simulink model "IEEE123_4subsystem"  (R2022b)
settings: Solver=ode4  StartTime=0.0  StopTime=inf  FixedStep=Ts  MaxStep=1e-4  RelTol=1e-3
PreLoadFcn:
  | Ts = 50e-6;
PostLoadFcn:
  | Ts = 50e-6;
InitFcn:
  | %%%%%%%%%%%%%%%%%%%%%%%%
  | % Simulation data for the IEEE 123 Node Test Feeder model
  | %%%%%%%%%%%%%%%%%%%%%%%
  | 
  | % miles/km
  | mi2km = 1.60934;
  | 
  | % feet to km
  | ft2km = 0.0003048;
  | 
  | % microsiemens to Farads
  | ms2F = 1/2/pi/60*1e-6;
  | 
  | %% Configuration 1 - series reactance - ohm/mile
  | 
  | R_1 = [0.4576 0.1560 0.1535;0.1560 0.4666 0.1580;0.1535 0.1580 0.4615];
  | X_1 = [1.0780 0.5017 0.3849;0.5017 1.0482 0.4236;0.3849 0.4236 1.0651];
  | 
  | % charging susceptance - microsiemens/mile
  | 
  | B_1 = [5.6765 -1.8319 -0.6982;-1.8319 5.9809 -1.1645;-0.6982 -1.1645 5.3971];
  | 
  | % convert for SPS
  | 
  | R_1 = R_1/mi2km;
  | 
  | Rs_1=(R_1(1,1)+R_1(2,2)+R_1(3,3))/3;
  | Rm_1=(R_1(1,2)+R_1(1,3)+R_1(2,3))/3;
  | R1_1=Rs_1-Rm_1;
  | R0_1=Rs_1+2*Rm_1;
  | 
  | L_1 = X_1/mi2km/2/pi/60;
  | 
  | Ls_1=(L_1(1,1)+L_1(2,2)+L_1(3,3))/3;
  | Lm_1=(L_1(1,2)+L_1(1,3)+L_1(2,3))/3;
  | L1_1=Ls_1-Lm_1;
  | L0_1=Ls_1+2*Lm_1;
  | 
  | C_1 = B_1/mi2km*ms2F;
  | 
  | Cs_1=(C_1(1,1)+C_1(2,2)+C_1(3,3))/3;
  | Cm_1=(C_1(1,2)+C_1(1,3)+C_1(2,3))/3;
  | C1_1=Cs_1-Cm_1;
  | C0_1=Cs_1+2*Cm_1;
  | 
  | 
  | %% Configuration 2 - series reactance - ohm/mile
  | 
  | R_2 = [0.4666 0.1580 0.1560;0.1580 0.4615 0.1535;0.1560 0.1535 0.4576];
  | X_2 = [1.0482 0.4236 0.5017;0.4236 1.0651 0.3849;0.5017 0.3849 1.0780];
  | 
  | % charging susceptance - microsiemens/mile
  | 
  | B_2 = [5.9809 -1.1645 -1.8319;-1.1645 5.3971 -0.6982;-1.8319 -0.6982 5.6765];
  | 
  | % convert for SPS
  | 
  | R_2 = R_2/mi2km;
  | 
  | Rs_2=(R_2(1,1)+R_2(2,2)+R_2(3,3))/3;
  | ... (+341 lines)
undefined symbols (not defined in the file): D1, Delta, find_system, I, Left, MOV_segment9, powergui, Right, type, V, X
libraries: spsGroundLib x242, spsThreePhaseVIMeasurementLib x134, spsSeriesRLCBranchLib x107, spsSeriesRLCLoadLib x83, spsPiSectionLineLib x61, spsThreePhasePISectionLineLib x60, spsVoltageMeasurementLib x52, spsDCVoltageSourceLib x36, ssn_lib x28, artemis x24, spsACCurrentSourceLib x18, spsOnDelayLib x18
(part 3 of 15)

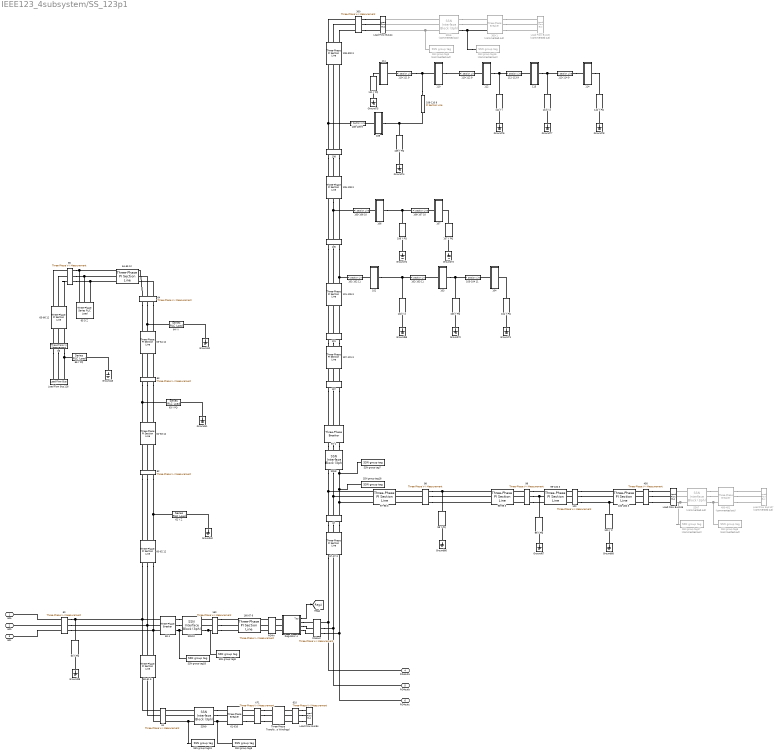
== system IEEE123_4subsystem/SS_123p1 ==
  100 : spsThreePhaseVIMeasurementLib/Three-Phase V-I Measurement  VoltageMeasurement=phase-to-ground  SetLabelV=on  LabelV=V100  Vpu=off  VpuLL=off  CurrentMeasurement=no  SetLabelI=on  LabelI=I65  Ipu=off  Pbase=100e6  Vbase=24900  OutputType=Complex  PhasorSimulation=off  PSBequivalent=0
  100 Y Z : spsSeriesRLCLoadLib/Series RLC Load  LConnTagsString=a  RConnTagsString=__new0  NominalVoltage=1.0*2401.78  NominalFrequency=60  ActivePower=40e3  InductivePower=20e3  CapacitivePower=0  Setx0=off  InitialVoltage=0  SetiL0=off  InitialCurrent=0  Measurements=None  LoadType=constant Z
  100-450 3 : spsThreePhasePISectionLineLib/Three-Phase PI Section Line  LConnTagsString=a|b|c  RConnTagsString=A|B|C  Length=800*ft2km  Frequency=60  Resistances=[R1_3 R0_3]  Inductances=[L1_3 L0_3]  Capacitances=[C1_3 C0_3]
  101 : spsThreePhaseVIMeasurementLib/Three-Phase V-I Measurement  VoltageMeasurement=phase-to-ground  SetLabelV=on  LabelV=V101  Vpu=off  VpuLL=off  CurrentMeasurement=no  SetLabelI=on  LabelI=I65  Ipu=off  Pbase=100e6  Vbase=24900  OutputType=Complex  PhasorSimulation=off  PSBequivalent=0
  101-102 11 : spsPiSectionLineLib/Pi Section Line  LConnTagsString=__new0  RConnTagsString=__new0  Phases=1  PiSections=1  Length=225*ft2km  Frequency=60  Resistance=R1_11  Inductance=L1_11  Capacitance=C1_11  SpecifyConductance=off  Conductance=0  Measurements=None  Measurements2=None
      settings: LibrarySourceBlock=sps_lib/Power Grid Elements/Pi Section Line
  101-105 3 : spsThreePhasePISectionLineLib/Three-Phase PI Section Line  LConnTagsString=a|b|c  RConnTagsString=A|B|C  Length=275*ft2km  Frequency=60  Resistances=[R1_3 R0_3]  Inductances=[L1_3 L0_3]  Capacitances=[C1_3 C0_3]
  102 : Subsystem
  102 Y Z : spsSeriesRLCLoadLib/Series RLC Load  LConnTagsString=a  RConnTagsString=__new0  NominalVoltage=1.0*2401.78  NominalFrequency=60  ActivePower=20e3  InductivePower=10e3  CapacitivePower=0  Setx0=off  InitialVoltage=0  SetiL0=off  InitialCurrent=0  Measurements=None  LoadType=constant Z
  102-103 11 : spsPiSectionLineLib/Pi Section Line  LConnTagsString=__new0  RConnTagsString=__new0  Phases=1  PiSections=1  Length=325*ft2km  Frequency=60  Resistance=R1_11  Inductance=L1_11  Capacitance=C1_11  SpecifyConductance=off  Conductance=0  Measurements=None  Measurements2=None
      settings: LibrarySourceBlock=sps_lib/Power Grid Elements/Pi Section Line
  103 : Subsystem
  103 Y PQ : spsSeriesRLCLoadLib/Series RLC Load  LConnTagsString=a  RConnTagsString=__new0  NominalVoltage=1.0*2401.78  NominalFrequency=60  ActivePower=40e3  InductivePower=20e3  CapacitivePower=0  Setx0=off  InitialVoltage=0  SetiL0=off  InitialCurrent=0  Measurements=None  LoadType=constant PQ
  103-104 11 : spsPiSectionLineLib/Pi Section Line  LConnTagsString=__new0  RConnTagsString=__new0  Phases=1  PiSections=1  Length=700*ft2km  Frequency=60  Resistance=R1_11  Inductance=L1_11  Capacitance=C1_11  SpecifyConductance=off  Conductance=0  Measurements=None  Measurements2=None
      settings: LibrarySourceBlock=sps_lib/Power Grid Elements/Pi Section Line
  104 : Subsystem
  104 Y PQ : spsSeriesRLCLoadLib/Series RLC Load  LConnTagsString=a  RConnTagsString=__new0  NominalVoltage=1.0*2401.78  NominalFrequency=60  ActivePower=40e3  InductivePower=20e3  CapacitivePower=0  Setx0=off  InitialVoltage=0  SetiL0=off  InitialCurrent=0  Measurements=None  LoadType=constant PQ
  105 : spsThreePhaseVIMeasurementLib/Three-Phase V-I Measurement  VoltageMeasurement=phase-to-ground  SetLabelV=on  LabelV=V105  Vpu=off  VpuLL=off  CurrentMeasurement=no  SetLabelI=on  LabelI=I65  Ipu=off  Pbase=100e6  Vbase=24900  OutputType=Complex  PhasorSimulation=off  PSBequivalent=0
  105-106 10 : spsPiSectionLineLib/Pi Section Line  LConnTagsString=__new0  RConnTagsString=__new0  Phases=1  PiSections=1  Length=225*ft2km  Frequency=60  Resistance=R1_10  Inductance=L1_10  Capacitance=C1_10  SpecifyConductance=off  Conductance=0  Measurements=None  Measurements2=None
      settings: LibrarySourceBlock=sps_lib/Power Grid Elements/Pi Section Line
  105-108 3 : spsThreePhasePISectionLineLib/Three-Phase PI Section Line  LConnTagsString=a|b|c  RConnTagsString=A|B|C  Length=325*ft2km  Frequency=60  Resistances=[R1_3 R0_3]  Inductances=[L1_3 L0_3]  Capacitances=[C1_3 C0_3]
  106 : Subsystem
  106 Y PQ : spsSeriesRLCLoadLib/Series RLC Load  LConnTagsString=a  RConnTagsString=__new0  NominalVoltage=1.0*2401.78  NominalFrequency=60  ActivePower=40e3  InductivePower=20e3  CapacitivePower=0  Setx0=off  InitialVoltage=0  SetiL0=off  InitialCurrent=0  Measurements=None  LoadType=constant PQ
  106-107 10 : spsPiSectionLineLib/Pi Section Line  LConnTagsString=__new0  RConnTagsString=__new0  Phases=1  PiSections=1  Length=575*ft2km  Frequency=60  Resistance=R1_10  Inductance=L1_10  Capacitance=C1_10  SpecifyConductance=off  Conductance=0  Measurements=None  Measurements2=None
      settings: LibrarySourceBlock=sps_lib/Power Grid Elements/Pi Section Line
  107 : Subsystem
  107 Y PQ : spsSeriesRLCLoadLib/Series RLC Load  LConnTagsString=a  RConnTagsString=__new0  NominalVoltage=1.0*2401.78  NominalFrequency=60  ActivePower=40e3  InductivePower=20e3  CapacitivePower=0  Setx0=off  InitialVoltage=0  SetiL0=off  InitialCurrent=0  Measurements=None  LoadType=constant PQ
  108 : spsThreePhaseVIMeasurementLib/Three-Phase V-I Measurement  VoltageMeasurement=phase-to-ground  SetLabelV=on  LabelV=V108  Vpu=off  VpuLL=off  CurrentMeasurement=no  SetLabelI=on  LabelI=I65  Ipu=off  Pbase=100e6  Vbase=24900  OutputType=Complex  PhasorSimulation=off  PSBequivalent=0
  108-109 9 : spsPiSectionLineLib/Pi Section Line  LConnTagsString=__new0  RConnTagsString=__new0  Phases=1  PiSections=1  Length=450*ft2km  Frequency=60  Resistance=R1_9  Inductance=L1_9  Capacitance=C1_9  SpecifyConductance=off  Conductance=0  Measurements=None  Measurements2=None
      settings: LibrarySourceBlock=sps_lib/Power Grid Elements/Pi Section Line
  108-300 3 : spsThreePhasePISectionLineLib/Three-Phase PI Section Line  LConnTagsString=a|b|c  RConnTagsString=A|B|C  Length=1000*ft2km  Frequency=60  Resistances=[R1_3 R0_3]  Inductances=[L1_3 L0_3]  Capacitances=[C1_3 C0_3]
  109 : Subsystem
  109 Y PQ : spsSeriesRLCLoadLib/Series RLC Load  LConnTagsString=a  RConnTagsString=__new0  NominalVoltage=1.0*2401.78  NominalFrequency=60  ActivePower=40e3  InductivePower=20e3  CapacitivePower=0  Setx0=off  InitialVoltage=0  SetiL0=off  InitialCurrent=0  Measurements=None  LoadType=constant PQ
  109-110 9 : spsPiSectionLineLib/Pi Section Line  LConnTagsString=__new0  RConnTagsString=__new0  Phases=1  PiSections=1  Length=300*ft2km  Frequency=60  Resistance=R1_9  Inductance=L1_9  Capacitance=C1_9  SpecifyConductance=off  Conductance=0  Measurements=None  Measurements2=None
      settings: LibrarySourceBlock=sps_lib/Power Grid Elements/Pi Section Line
  110 : Subsystem
  110-111 9 : spsPiSectionLineLib/Pi Section Line  LConnTagsString=__new0  RConnTagsString=__new0  Phases=1  PiSections=1  Length=575*ft2km  Frequency=60  Resistance=R1_9  Inductance=L1_9  Capacitance=C1_9  SpecifyConductance=off  Conductance=0  Measurements=None  Measurements2=None
      settings: LibrarySourceBlock=sps_lib/Power Grid Elements/Pi Section Line
  110-112 9 : spsPiSectionLineLib/Pi Section Line  LConnTagsString=__new0  RConnTagsString=__new0  Phases=1  PiSections=1  Length=125*ft2km  Frequency=60  Resistance=R1_9  Inductance=L1_9  Capacitance=C1_9  SpecifyConductance=off  Conductance=0  Measurements=None  Measurements2=None
      settings: LibrarySourceBlock=sps_lib/Power Grid Elements/Pi Section Line
  111 : Subsystem
  111 Y PQ : spsSeriesRLCLoadLib/Series RLC Load  LConnTagsString=a  RConnTagsString=__new0  NominalVoltage=1.0*2401.78  NominalFrequency=60  ActivePower=20e3  InductivePower=10e3  CapacitivePower=0  Setx0=off  InitialVoltage=0  SetiL0=off  InitialCurrent=0  Measurements=None  LoadType=constant PQ
  112 : Subsystem
  112 Y I : spsSeriesRLCLoadLib/Series RLC Load  LConnTagsString=a  RConnTagsString=__new0  NominalVoltage=1.0*2401.78  NominalFrequency=60  ActivePower=20e3  InductivePower=10e3  CapacitivePower=0  Setx0=off  InitialVoltage=0  SetiL0=off  InitialCurrent=0  Measurements=None  LoadType=constant I
  112-113 9 : spsPiSectionLineLib/Pi Section Line  LConnTagsString=__new0  RConnTagsString=__new0  Phases=1  PiSections=1  Length=525*ft2km  Frequency=60  Resistance=R1_9  Inductance=L1_9  Capacitance=C1_9  SpecifyConductance=off  Conductance=0  Measurements=None  Measurements2=None
      settings: LibrarySourceBlock=sps_lib/Power Grid Elements/Pi Section Line
  113 : Subsystem
  113 Y Z : spsSeriesRLCLoadLib/Series RLC Load  LConnTagsString=a  RConnTagsString=__new0  NominalVoltage=1.0*2401.78  NominalFrequency=60  ActivePower=40e3  InductivePower=20e3  CapacitivePower=0  Setx0=off  InitialVoltage=0  SetiL0=off  InitialCurrent=0  Measurements=None  LoadType=constant PQ
  113-114 9 : spsPiSectionLineLib/Pi Section Line  LConnTagsString=__new0  RConnTagsString=__new0  Phases=1  PiSections=1  Length=325*ft2km  Frequency=60  Resistance=R1_9  Inductance=L1_9  Capacitance=C1_9  SpecifyConductance=off  Conductance=0  Measurements=None  Measurements2=None
      settings: LibrarySourceBlock=sps_lib/Power Grid Elements/Pi Section Line
  114 : Subsystem
  142 Y PQ : spsSeriesRLCLoadLib/Series RLC Load  LConnTagsString=a  RConnTagsString=__new0  NominalVoltage=1.0*2401.78  NominalFrequency=60  ActivePower=20e3  InductivePower=10e3  CapacitivePower=0  Setx0=off  InitialVoltage=0  SetiL0=off  InitialCurrent=0  Measurements=None  LoadType=constant PQ
  160 : spsThreePhaseVIMeasurementLib/Three-Phase V-I Measurement  VoltageMeasurement=phase-to-ground  SetLabelV=on  LabelV=V160  Vpu=off  VpuLL=off  CurrentMeasurement=no  SetLabelI=on  LabelI=I160  Ipu=off  Pbase=100e6  Vbase=24900  OutputType=Complex  PhasorSimulation=off  PSBequivalent=0
  160 67 6 : spsThreePhasePISectionLineLib/Three-Phase PI Section Line  LConnTagsString=a|b|c  RConnTagsString=A|B|C  Length=350*ft2km  Frequency=60  Resistances=[R1_6 R0_6]  Inductances=[L1_6 L0_6]  Capacitances=[C1_6 C0_6]
  197 : spsThreePhaseVIMeasurementLib/Three-Phase V-I Measurement  VoltageMeasurement=phase-to-ground  SetLabelV=on  LabelV=V197  Vpu=off  VpuLL=off  CurrentMeasurement=no  SetLabelI=on  LabelI=I65  Ipu=off  Pbase=100e6  Vbase=24900  OutputType=Complex  PhasorSimulation=off  PSBequivalent=0
  197-101 3 : spsThreePhasePISectionLineLib/Three-Phase PI Section Line  LConnTagsString=a|b|c  RConnTagsString=A|B|C  Length=250*ft2km  Frequency=60  Resistances=[R1_3 R0_3]  Inductances=[L1_3 L0_3]  Capacitances=[C1_3 C0_3]
  300 : spsThreePhaseVIMeasurementLib/Three-Phase V-I Measurement  VoltageMeasurement=phase-to-ground  SetLabelV=on  LabelV=V300  Vpu=off  VpuLL=off  CurrentMeasurement=no  SetLabelI=on  LabelI=I65  Ipu=off  Pbase=100e6  Vbase=24900  OutputType=Complex  PhasorSimulation=off  PSBequivalent=0
  300-1 : spsThreePhaseBreakerLib/Three-Phase Breaker  Commented=on  InitialState=open  SwitchA=on  SwitchB=on  SwitchC=on  SwitchTimes="[1/60  5/60]"  External=off  BreakerResistance=0.01  SnubberResistance=1e6  SnubberCapacitance=inf  Measurements=None
  450 : spsThreePhaseVIMeasurementLib/Three-Phase V-I Measurement  VoltageMeasurement=phase-to-ground  SetLabelV=on  LabelV=V450  Vpu=off  VpuLL=off  CurrentMeasurement=no  SetLabelI=on  LabelI=I65  Ipu=off  Pbase=100e6  Vbase=24900  OutputType=Complex  PhasorSimulation=off  PSBequivalent=0
  450-451 : spsThreePhaseBreakerLib/Three-Phase Breaker  Commented=on  InitialState=open  SwitchA=on  SwitchB=on  SwitchC=on  SwitchTimes="[1/60  5/60]"  External=off  BreakerResistance=0.01  SnubberResistance=1e6  SnubberCapacitance=inf  Measurements=None
  60 : spsThreePhaseVIMeasurementLib/Three-Phase V-I Measurement  VoltageMeasurement=phase-to-ground  SetLabelV=on  LabelV=V60  Vpu=off  VpuLL=off  CurrentMeasurement=yes  SetLabelI=on  LabelI=I60  Ipu=off  Pbase=100e6  Vbase=24900  OutputType=Complex  PhasorSimulation=off  PSBequivalent=0
  60 Y PQ : spsSeriesRLCLoadLib/Series RLC Load  LConnTagsString=a  RConnTagsString=__new0  NominalVoltage=1.0*2401.78  NominalFrequency=60  ActivePower=20e3  InductivePower=10e3  CapacitivePower=0  Setx0=off  InitialVoltage=0  SetiL0=off  InitialCurrent=0  Measurements=None  LoadType=constant PQ
  60-1 : spsThreePhaseBreakerLib/Three-Phase Breaker  InitialState=closed  SwitchA=on  SwitchB=on  SwitchC=on  SwitchTimes="[1/60  5/60]"  External=off  BreakerResistance=0.01  SnubberResistance=1e6  SnubberCapacitance=inf  Measurements=None
  60-61 5 : spsThreePhasePISectionLineLib/Three-Phase PI Section Line  LConnTagsString=a|b|c  RConnTagsString=A|B|C  Length=550*ft2km  Frequency=60  Resistances=[R1_5 R0_5]  Inductances=[L1_5 L0_5]  Capacitances=[C1_5 C0_5]
  60-62 12 : spsThreePhasePISectionLineLib/Three-Phase PI Section Line  LConnTagsString=a|b|c  RConnTagsString=A|B|C  Length=250*ft2km  Frequency=60  Resistances=[R1_12 R0_12]  Inductances=[L1_12 L0_12]  Capacitances=[C1_12 C0_12]
  61 : spsThreePhaseVIMeasurementLib/Three-Phase V-I Measurement  VoltageMeasurement=phase-to-ground  SetLabelV=on  LabelV=V61  Vpu=off  VpuLL=off  CurrentMeasurement=no  SetLabelI=on  LabelI=I65  Ipu=off  Pbase=100e6  Vbase=24900  OutputType=Complex  PhasorSimulation=off  PSBequivalent=0
  61-610 : spsThreePhaseBreakerLib/Three-Phase Breaker  InitialState=closed  SwitchA=on  SwitchB=on  SwitchC=on  SwitchTimes="[1/60  5/60]"  External=off  BreakerResistance=0.01  SnubberResistance=1e6  SnubberCapacitance=inf  Measurements=None
  610 : spsThreePhaseVIMeasurementLib/Three-Phase V-I Measurement  VoltageMeasurement=phase-to-phase  SetLabelV=on  LabelV=V610  Vpu=off  VpuLL=off  CurrentMeasurement=no  SetLabelI=on  LabelI=I65  Ipu=off  Pbase=100e6  Vbase=24900  OutputType=Complex  PhasorSimulation=off  PSBequivalent=0
  62 : spsThreePhaseVIMeasurementLib/Three-Phase V-I Measurement  VoltageMeasurement=phase-to-ground  SetLabelV=on  LabelV=V62  Vpu=off  VpuLL=off  CurrentMeasurement=no  SetLabelI=on  LabelI=I65  Ipu=off  Pbase=100e6  Vbase=24900  OutputType=Complex  PhasorSimulation=off  PSBequivalent=0
  62 Y Z : spsSeriesRLCLoadLib/Series RLC Load  LConnTagsString=a  RConnTagsString=__new0  NominalVoltage=1.0*2401.78  NominalFrequency=60  ActivePower=40e3  InductivePower=20e3  CapacitivePower=0  Setx0=off  InitialVoltage=0  SetiL0=off  InitialCurrent=0  Measurements=None  LoadType=constant Z
  62-63 12 : spsThreePhasePISectionLineLib/Three-Phase PI Section Line  LConnTagsString=a|b|c  RConnTagsString=A|B|C  Length=175*ft2km  Frequency=60  Resistances=[R1_12 R0_12]  Inductances=[L1_12 L0_12]  Capacitances=[C1_12 C0_12]
  63 : spsThreePhaseVIMeasurementLib/Three-Phase V-I Measurement  VoltageMeasurement=phase-to-ground  SetLabelV=on  LabelV=V63  Vpu=off  VpuLL=off  CurrentMeasurement=no  SetLabelI=on  LabelI=I65  Ipu=off  Pbase=100e6  Vbase=24900  OutputType=Complex  PhasorSimulation=off  PSBequivalent=0
  63 Y PQ : spsSeriesRLCLoadLib/Series RLC Load  LConnTagsString=a  RConnTagsString=__new0  NominalVoltage=1.0*2401.78  NominalFrequency=60  ActivePower=40e3  InductivePower=20e3  CapacitivePower=0  Setx0=off  InitialVoltage=0  SetiL0=off  InitialCurrent=0  Measurements=None  LoadType=constant PQ
  63-64 12 : spsThreePhasePISectionLineLib/Three-Phase PI Section Line  LConnTagsString=a|b|c  RConnTagsString=A|B|C  Length=350*ft2km  Frequency=60  Resistances=[R1_12 R0_12]  Inductances=[L1_12 L0_12]  Capacitances=[C1_12 C0_12]
  64 : spsThreePhaseVIMeasurementLib/Three-Phase V-I Measurement  VoltageMeasurement=phase-to-ground  SetLabelV=on  LabelV=V64  Vpu=off  VpuLL=off  CurrentMeasurement=no  SetLabelI=on  LabelI=I65  Ipu=off  Pbase=100e6  Vbase=24900  OutputType=Complex  PhasorSimulation=off  PSBequivalent=0
  64 Y I : spsSeriesRLCLoadLib/Series RLC Load  LConnTagsString=a  RConnTagsString=__new0  NominalVoltage=1.0*2401.78  NominalFrequency=60  ActivePower=75e3  InductivePower=35e3  CapacitivePower=0  Setx0=off  InitialVoltage=0  SetiL0=off  InitialCurrent=0  Measurements=None  LoadType=constant I
  64-65 12 : spsThreePhasePISectionLineLib/Three-Phase PI Section Line  LConnTagsString=a|b|c  RConnTagsString=A|B|C  Length=425*ft2km  Frequency=60  Resistances=[R1_12 R0_12]  Inductances=[L1_12 L0_12]  Capacitances=[C1_12 C0_12]
  65 : spsThreePhaseVIMeasurementLib/Three-Phase V-I Measurement  VoltageMeasurement=phase-to-ground  SetLabelV=on  LabelV=V65  Vpu=off  VpuLL=off  CurrentMeasurement=yes  SetLabelI=on  LabelI=I65  Ipu=off  Pbase=100e6  Vbase=24900  OutputType=Complex  PhasorSimulation=off  PSBequivalent=0
  65 D Z : spsThreePhaseSeriesRLCLoadLib/Three-Phase Series RLC Load  LConnTagsString=A|B|C  Configuration=Delta  NominalVoltage=120e3  Vabc=[ 1.0 1.0 1.0]*2401.78  Vabcp=[ 1.0 1.0 1.0]*4160  NominalFrequency=60  UnbalancedPower=on  ActivePower=1e+006  InductivePower=0  CapacitivePower=0  Pabc="[17 66  117]*1e3/2"  QLabc="[10 38  68]*1e3/2"  QCabc=[0 0 0]  Pabcp=[35 35 70]*1e3  QLabcp=[25 25 50]*1e3  QCabcp=[0 0 0]  Measurements=None  LoadType=constant Z
  65-66 12 : spsThreePhasePISectionLineLib/Three-Phase PI Section Line  LConnTagsString=a|b|c  RConnTagsString=A|B|C  Length=325*ft2km  Frequency=60  Resistances=[R1_12 R0_12]  Inductances=[L1_12 L0_12]  Capacitances=[C1_12 C0_12]
  66 : spsThreePhaseVIMeasurementLib/Three-Phase V-I Measurement  VoltageMeasurement=phase-to-ground  SetLabelV=on  LabelV=V66  Vpu=off  VpuLL=off  CurrentMeasurement=no  SetLabelI=on  LabelI=I65  Ipu=off  Pbase=100e6  Vbase=24900  OutputType=Complex  PhasorSimulation=off  PSBequivalent=0
  66 Y PQ : spsSeriesRLCLoadLib/Series RLC Load  LConnTagsString=a  RConnTagsString=__new0  NominalVoltage=1.0*2401.78  NominalFrequency=60  ActivePower=75e3  InductivePower=35e3  CapacitivePower=0  Setx0=off  InitialVoltage=0  SetiL0=off  InitialCurrent=0  Measurements=None  LoadType=constant PQ
  67-97 3 : spsThreePhasePISectionLineLib/Three-Phase PI Section Line  LConnTagsString=a|b|c  RConnTagsString=A|B|C  Length=250*ft2km  Frequency=60  Resistances=[R1_3 R0_3]  Inductances=[L1_3 L0_3]  Capacitances=[C1_3 C0_3]
  97 : spsThreePhaseVIMeasurementLib/Three-Phase V-I Measurement  VoltageMeasurement=phase-to-ground  SetLabelV=on  LabelV=V97  Vpu=off  VpuLL=off  CurrentMeasurement=yes  SetLabelI=on  LabelI=I97  Ipu=off  Pbase=100e6  Vbase=24900  OutputType=Complex  PhasorSimulation=off  PSBequivalent=0
  97-1 : spsThreePhaseBreakerLib/Three-Phase Breaker  InitialState=closed  SwitchA=on  SwitchB=on  SwitchC=on  SwitchTimes="[1/60  5/60]"  External=off  BreakerResistance=0.01  SnubberResistance=1e6  SnubberCapacitance=inf  Measurements=None
  97-98 3 : spsThreePhasePISectionLineLib/Three-Phase PI Section Line  LConnTagsString=a|b|c  RConnTagsString=A|B|C  Length=275*ft2km  Frequency=60  Resistances=[R1_3 R0_3]  Inductances=[L1_3 L0_3]  Capacitances=[C1_3 C0_3]
  98 : spsThreePhaseVIMeasurementLib/Three-Phase V-I Measurement  VoltageMeasurement=phase-to-ground  SetLabelV=on  LabelV=V98  Vpu=off  VpuLL=off  CurrentMeasurement=yes  SetLabelI=on  LabelI=I98  Ipu=off  Pbase=100e6  Vbase=24900  OutputType=Complex  PhasorSimulation=off  PSBequivalent=0
  98 Y PQ : spsSeriesRLCLoadLib/Series RLC Load  LConnTagsString=a  RConnTagsString=__new0  NominalVoltage=1.0*2401.78  NominalFrequency=60  ActivePower=40e3  InductivePower=20e3  CapacitivePower=0  Setx0=off  InitialVoltage=0  SetiL0=off  InitialCurrent=0  Measurements=None  LoadType=constant PQ
  98-99 3 : spsThreePhasePISectionLineLib/Three-Phase PI Section Line  LConnTagsString=a|b|c  RConnTagsString=A|B|C  Length=550*ft2km  Frequency=60  Resistances=[R1_3 R0_3]  Inductances=[L1_3 L0_3]  Capacitances=[C1_3 C0_3]
  99 : spsThreePhaseVIMeasurementLib/Three-Phase V-I Measurement  VoltageMeasurement=phase-to-ground  SetLabelV=on  LabelV=V99  Vpu=off  VpuLL=off  CurrentMeasurement=no  SetLabelI=on  LabelI=I65  Ipu=off  Pbase=100e6  Vbase=24900  OutputType=Complex  PhasorSimulation=off  PSBequivalent=0
  99 Y PQ : spsSeriesRLCLoadLib/Series RLC Load  LConnTagsString=a  RConnTagsString=__new0  NominalVoltage=1.0*2401.78  NominalFrequency=60  ActivePower=40e3  InductivePower=20e3  CapacitivePower=0  Setx0=off  InitialVoltage=0  SetiL0=off  InitialCurrent=0  Measurements=None  LoadType=constant PQ
  99-100 3 : spsThreePhasePISectionLineLib/Three-Phase PI Section Line  LConnTagsString=a|b|c  RConnTagsString=A|B|C  Length=300*ft2km  Frequency=60  Resistances=[R1_3 R0_3]  Inductances=[L1_3 L0_3]  Capacitances=[C1_3 C0_3]
  Ground{39..43,66..78} (18 alike) : spsGroundLib/Ground  LConnTagsString=a
  Load Flow Bus106 : spsLoadFlowBusLib/Load Flow Bus  LConnTagsString=a|b|c  RConnTagsString=a|b|c  Phases=ABC  Connectors=on both sides  ID=450  Vbase=4160/sqrt(3)  Vref=[1.0 1.0 1.0]  Vangle=[0 -120 120]  VLF=1  VLFb=1  VLFc=1  angleLF=0  angleLFb=0  angleLFc=0
  Load Flow Bus107 : spsLoadFlowBusLib/Load Flow Bus  Commented=on  LConnTagsString=a|b|c  Phases=ABC  Connectors=on one side  ID=451  Vbase=4160/sqrt(3)  Vref=[1.0 1.0 1.0]  Vangle=[0 -120 120]  VLF=1  VLFb=1  VLFc=1  angleLF=0  angleLFb=0  angleLFc=0
  Load Flow Bus128 : spsLoadFlowBusLib/Load Flow Bus  LConnTagsString=a|b|c  Phases=ABC  Connectors=on one side  ID=66  Vbase=4160/sqrt(3)  Vref=[1.0 1.0 1.0]  Vangle=[0 -120 120]  VLF=1  VLFb=1  VLFc=1  angleLF=0  angleLFb=0  angleLFc=0
  Load Flow Bus44 : spsLoadFlowBusLib/Load Flow Bus  LConnTagsString=a|b|c  RConnTagsString=a|b|c  Phases=ABC  Connectors=on both sides  ID=300  Vbase=4160/sqrt(3)  Vref=[1.0 1.0 1.0]  Vangle=[0 -120 120]  VLF=1  VLFb=1  VLFc=1  angleLF=0  angleLFb=0  angleLFc=0
  Load Flow Bus45 : spsLoadFlowBusLib/Load Flow Bus  Commented=on  LConnTagsString=a|b|c  Phases=ABC  Connectors=on one side  ID=350  Vbase=4160/sqrt(3)  Vref=[1.0 1.0 1.0]  Vangle=[0 -120 120]  VLF=1  VLFb=1  VLFc=1  angleLF=0  angleLFb=0  angleLFc=0
  Load Flow Bus84 : spsLoadFlowBusLib/Load Flow Bus  LConnTagsString=a|b|c  Phases=ABC  Connectors=on one side  ID=610  Vbase=480/sqrt(3)  Vref=[1.0 1.0 1.0]  Vangle=[0 -120 120]  VLF=1  VLFb=1  VLFc=1  angleLF=0  angleLFb=0  angleLFc=0
  RG4in : spsThreePhaseVIMeasurementLib/Three-Phase V-I Measurement  VoltageMeasurement=phase-to-ground  SetLabelV=on  LabelV=RG4in  Vpu=off  VpuLL=off  CurrentMeasurement=yes  SetLabelI=on  LabelI=IRG4in  Ipu=off  Pbase=100e6  Vbase=24900  OutputType=Complex  PhasorSimulation=off  PSBequivalent=0
  RG4out : spsThreePhaseVIMeasurementLib/Three-Phase V-I Measurement  VoltageMeasurement=phase-to-ground  SetLabelV=on  LabelV=RG4out  Vpu=off  VpuLL=off  CurrentMeasurement=no  SetLabelI=on  LabelI=I800  Ipu=off  Pbase=100e6  Vbase=24900  OutputType=Complex  PhasorSimulation=off  PSBequivalent=0
  Regulator 4 : Subsystem
  SSN group tag16 : artemis/SSN/SSN group tag  Commented=on  ssn_group_tag=ssn6b
  SSN group tag17 : artemis/SSN/SSN group tag  Commented=on  ssn_group_tag=ssn7a
  SSN group tag18 : artemis/SSN/SSN group tag  ssn_group_tag=ssn8a
  SSN group tag19 : artemis/SSN/SSN group tag  ssn_group_tag=ssn9a
  SSN group tag20 : artemis/SSN/SSN group tag  ssn_group_tag=ssn10a
  SSN group tag5 : artemis/SSN/SSN group tag  Commented=on  ssn_group_tag=ssn6a
  SSN group tag6 : artemis/SSN/SSN group tag  Commented=on  ssn_group_tag=ssn7b
  SSN group tag7 : artemis/SSN/SSN group tag  ssn_group_tag=ssn8b
  SSN group tag8 : artemis/SSN/SSN group tag  ssn_group_tag=ssn9b
  SSN group tag9 : artemis/SSN/SSN group tag  ssn_group_tag=ssn10b
  SSN10 : ssn_lib/SSN Interface Block (3ph)  nb_phase=3  nb_port=2  p1_type=I-type(Left)  p2_type=I-type(Right)  p3_type=V-type(Left)  p4_type=V-type(Left)  p5_type=V-type(Left)  p6_type=V-type(Left)  p7_type=V-type(Left)  p8_type=V-type(Left)  p9_type=V-type(Left)  p10_type=V-type(Left)  p11_type=V-type(Left)  p12_type=V-type(Left)  p13_type=V-type(Left)  p14_type=V-type(Left)  p15_type=V-type(Left)  p16_type=V-type(Left)  I_port_shunt_resistance=1e9
  SSN6 : ssn_lib/SSN Interface Block (3ph)  Commented=on  nb_phase=3  nb_port=2  p1_type=I-type(Left)  p2_type=I-type(Right)  p3_type=V-type(Left)  p4_type=V-type(Left)  p5_type=V-type(Left)  p6_type=V-type(Left)  p7_type=V-type(Left)  p8_type=V-type(Left)  p9_type=V-type(Left)  p10_type=V-type(Left)  p11_type=V-type(Left)  p12_type=V-type(Left)  p13_type=V-type(Left)  p14_type=V-type(Left)  p15_type=V-type(Left)  p16_type=V-type(Left)  I_port_shunt_resistance=1e9
  SSN7 : ssn_lib/SSN Interface Block (3ph)  Commented=on  nb_phase=3  nb_port=2  p1_type=I-type(Left)  p2_type=I-type(Right)  p3_type=V-type(Left)  p4_type=V-type(Left)  p5_type=V-type(Left)  p6_type=V-type(Left)  p7_type=V-type(Left)  p8_type=V-type(Left)  p9_type=V-type(Left)  p10_type=V-type(Left)  p11_type=V-type(Left)  p12_type=V-type(Left)  p13_type=V-type(Left)  p14_type=V-type(Left)  p15_type=V-type(Left)  p16_type=V-type(Left)  I_port_shunt_resistance=1e9
  SSN8 : ssn_lib/SSN Interface Block (3ph)  nb_phase=3  nb_port=2  p1_type=I-type(Left)  p2_type=I-type(Right)  p3_type=V-type(Left)  p4_type=V-type(Left)  p5_type=V-type(Left)  p6_type=V-type(Left)  p7_type=V-type(Left)  p8_type=V-type(Left)  p9_type=V-type(Left)  p10_type=V-type(Left)  p11_type=V-type(Left)  p12_type=V-type(Left)  p13_type=V-type(Left)  p14_type=V-type(Left)  p15_type=V-type(Left)  p16_type=V-type(Left)  I_port_shunt_resistance=1e9
  SSN9 : ssn_lib/SSN Interface Block (3ph)  nb_phase=3  nb_port=2  p1_type=I-type(Left)  p2_type=I-type(Right)  p3_type=V-type(Left)  p4_type=V-type(Left)  p5_type=V-type(Left)  p6_type=V-type(Left)  p7_type=V-type(Left)  p8_type=V-type(Left)  p9_type=V-type(Left)  p10_type=V-type(Left)  p11_type=V-type(Left)  p12_type=V-type(Left)  p13_type=V-type(Left)  p14_type=V-type(Left)  p15_type=V-type(Left)  p16_type=V-type(Left)  I_port_shunt_resistance=1e9
  Three-Phase Transformer (Two Windings) : spsThreePhaseTransformerTwoWindingsLib/Three-Phase Transformer (Two Windings)  Winding1Connection=Delta (D1)  Winding2Connection=Delta (D1)  CoreType=Three single-phase transformers  SetSaturation=off  Hysteresis=off  DataFile='hysteresis'  SetInitialFlux=off  Measurements=None  UNITS=pu  NominalPower=[ 500e3 , 60 ]  Winding1=[4160 0.0127 0.0272]  Winding2=[480 0.0127 0.0272]  Rm=500  Lm=500  L0=0.5  Saturation=[ 0,0 ; 0.0024,1.2 ; 1.0,1.52 ]  InitialFluxes=[ 0.8 , -0.8 , 0.7 ]  BreakLoop=off  DiscreteSolver=Trapezoidal iterative  DataType=off  TransfoNumber=1
  XF1 : spsThreePhaseVIMeasurementLib/Three-Phase V-I Measurement  VoltageMeasurement=phase-to-ground  SetLabelV=on  LabelV=XF1  Vpu=off  VpuLL=off  CurrentMeasurement=no  SetLabelI=on  LabelI=I65  Ipu=off  Pbase=100e6  Vbase=24900  OutputType=Complex  PhasorSimulation=off  PSBequivalent=0
  60a : PMIOPort  Side=Left
  60b : PMIOPort  Port=2  Side=Left
  60c : PMIOPort  Port=3  Side=Left
  RG4outa : PMIOPort  Port=4  Side=Right
  RG4outb : PMIOPort  Port=5  Side=Right
  RG4outc : PMIOPort  Port=6  Side=Right
  tag scope: Reg4=global
  wires:
  Regulator 4/1(Tap) -> [Reg4]
  connections:
  105/LConn1 -- 101-105 3/RConn1
  64 Y I/LConn1 -- 64/LConn2 -- 63-64 12/RConn2
  Ground70/LConn1 -- 103 Y PQ/RConn1
  110/RConn1 -- 110-112 9/LConn1
  97/LConn2 -- 67-97 3/RConn2
  65/RConn1 -- 65-66 12/LConn1
  105-108 3/LConn2 -- 105/RConn2 -- 105-106 10/LConn1
  100 Y Z/LConn1 -- 100/RConn3 -- 100-450 3/LConn3
  SSN7/RConn3 -- SSN group tag6/LConn1 -- 450-451/LConn3
  63/LConn2 -- 62-63 12/RConn2
  60/RConn2 -- 60b/RConn1
  60-61 5/LConn3 -- 60/LConn3 -- 60-1/LConn3 -- 60-62 12/LConn3
  Ground40/LConn1 -- 62 Y Z/RConn1
  99/RConn1 -- 99-100 3/LConn1
  60 Y PQ/LConn1 -- 60/LConn1 -- 60-1/LConn1 -- 60-61 5/LConn1 -- 60-62 12/LConn1
  108/LConn3 -- 105-108 3/RConn3
  62 Y Z/LConn1 -- 62/LConn3 -- 60-62 12/RConn3
  62/RConn2 -- 62-63 12/LConn2
  109-110 9/RConn1 -- 110/LConn1 -- 110-111 9/RConn1
  Ground41/LConn1 -- 63 Y PQ/RConn1
  197/LConn1 -- 97-1/RConn1
  SSN7/LConn2 -- Load Flow Bus106/RConn2
  111/RConn1 -- 111 Y PQ/LConn1
  97-1/LConn2 -- SSN8/LConn2
  61/LConn2 -- 60-61 5/RConn2
  61/LConn3 -- 60-61 5/RConn3
  300/LConn2 -- 108-300 3/RConn2
  66 Y PQ/LConn1 -- Load Flow Bus128/LConn3 -- 66/RConn3
  108/RConn3 -- 108-300 3/LConn3
  64/RConn3 -- 64-65 12/LConn3
  SSN group tag9/LConn1 -- 160/LConn3 -- SSN10/RConn3
  108/LConn2 -- 105-108 3/RConn2
  Ground66/LConn1 -- 98 Y PQ/RConn1
  Ground71/LConn1 -- 104 Y PQ/RConn1
  XF1/RConn1 -- Three-Phase Transformer (Two Windings)/LConn1
  Ground69/LConn1 -- 102 Y Z/RConn1
  SSN7/LConn3 -- SSN group tag17/LConn1 -- Load Flow Bus106/RConn3
  97/LConn3 -- 67-97 3/RConn3
  97-98 3/LConn2 -- 97/RConn2 -- SSN8/RConn2
  160/LConn2 -- SSN10/RConn2
  SSN group tag5/LConn1 -- SSN6/LConn3 -- Load Flow Bus44/RConn3
  Ground39/LConn1 -- 60 Y PQ/RConn1
  Ground76/LConn1 -- 112 Y I/RConn1
  65 D Z/LConn2 -- 64-65 12/RConn2 -- 65/LConn2
  101/LConn3 -- 197-101 3/RConn3
  Ground42/LConn1 -- 64 Y I/RConn1
  450-451/RConn1 -- Load Flow Bus107/LConn1
  Ground77/LConn1 -- 113 Y Z/RConn1
  62/LConn2 -- 60-62 12/RConn2
  108/RConn2 -- 108-300 3/LConn2
  63 Y PQ/LConn1 -- 63/LConn1 -- 62-63 12/RConn1
  Ground67/LConn1 -- 99 Y PQ/RConn1
  450/RConn2 -- Load Flow Bus106/LConn2
  SSN7/RConn2 -- 450-451/LConn2
  64/LConn1 -- 63-64 12/RConn1
  101/LConn1 -- 197-101 3/RConn1
  SSN6/LConn2 -- Load Flow Bus44/RConn2
  RG4in/LConn1 -- 160 67 6/RConn1
  SSN6/LConn1 -- Load Flow Bus44/RConn1
  112/LConn1 -- 110-112 9/RConn1
  63/RConn3 -- 63-64 12/LConn3
  101/LConn2 -- 197-101 3/RConn2
  103 Y PQ/LConn1 -- 103/RConn1 -- 103-104 11/LConn1
  67-97 3/LConn3 -- RG4out/RConn3 -- RG4outc/RConn1
  97/LConn1 -- 67-97 3/RConn1
  113/LConn1 -- 112-113 9/RConn1
  99/LConn2 -- 98-99 3/RConn2
  SSN8/RConn3 -- SSN group tag7/LConn1 -- SSN group tag18/LConn1 -- 97/RConn3 -- 97-98 3/LConn3
  101-102 11/LConn1 -- 105/LConn3 -- 101-105 3/RConn3
  Ground43/LConn1 -- 66 Y PQ/RConn1
  65 D Z/LConn3 -- 64-65 12/RConn3 -- 65/LConn3
  300/RConn3 -- Load Flow Bus44/LConn3
  SSN9/RConn3 -- SSN group tag8/LConn1 -- 61-610/LConn3
  197/RConn3 -- 197-101 3/LConn3
  62/LConn1 -- 60-62 12/RConn1
  101/RConn2 -- 101-105 3/LConn2
  450-451/RConn3 -- Load Flow Bus107/LConn3
  103/LConn1 -- 102-103 11/RConn1
  SSN9/RConn2 -- 61-610/LConn2
  101/RConn3 -- 101-105 3/LConn3
  106/LConn1 -- 105-106 10/RConn1
  104 Y PQ/LConn1 -- 104/RConn1
  65/RConn2 -- 65-66 12/LConn2
  63/RConn1 -- 63-64 12/LConn1
  63/RConn2 -- 63-64 12/LConn2
  300/LConn1 -- 108-300 3/RConn1
  60-61 5/LConn2 -- 60/LConn2 -- 60-1/LConn2 -- 60-62 12/LConn2
  99 Y PQ/LConn1 -- 99/RConn2 -- 99-100 3/LConn2
  64/RConn2 -- 64-65 12/LConn2
  62/RConn1 -- 62-63 12/LConn1
  SSN9/RConn1 -- 61-610/LConn1
  RG4out/RConn2 -- 67-97 3/LConn2 -- RG4outb/RConn1
  98/LConn3 -- 97-98 3/RConn3
  XF1/RConn3 -- Three-Phase Transformer (Two Windings)/LConn3
  160/RConn3 -- 160 67 6/LConn3
  101/RConn1 -- 101-105 3/LConn1
  98/RConn2 -- 98-99 3/LConn2
  610/LConn1 -- Three-Phase Transformer (Two Windings)/RConn1
  98/RConn3 -- 98-99 3/LConn3
  100/LConn3 -- 99-100 3/RConn3
  SSN group tag16/LConn1 -- SSN6/RConn3 -- 300-1/LConn3
  62/RConn3 -- 62-63 12/LConn3
  450/LConn2 -- 100-450 3/RConn2
  Ground75/LConn1 -- 111 Y PQ/RConn1
  100/RConn1 -- 100-450 3/LConn1
  100/LConn1 -- 99-100 3/RConn1
  197/RConn1 -- 197-101 3/LConn1
  97-98 3/LConn1 -- 97/RConn1 -- SSN8/RConn1
  65 D Z/LConn1 -- 64-65 12/RConn1 -- 65/LConn1
  60-1/RConn1 -- SSN10/LConn1
  99/LConn3 -- 98-99 3/RConn3
  108-109 9/LConn1 -- 108/RConn1 -- 108-300 3/LConn1
  105/LConn2 -- 101-105 3/RConn2
  102-103 11/LConn1 -- 102/RConn1 -- 102 Y Z/LConn1
  SSN10/LConn3 -- SSN group tag20/LConn1 -- 60-1/RConn3
  197/LConn3 -- 97-1/RConn3
  100/RConn2 -- 100-450 3/LConn2
  Ground73/LConn1 -- 107 Y PQ/RConn1
  Regulator 4/RConn1 -- RG4out/LConn1
  108/LConn1 -- 105-108 3/RConn1
  300-1/RConn2 -- Load Flow Bus45/LConn2
  109-110 9/LConn1 -- 109/RConn1 -- 109 Y PQ/LConn1
  Regulator 4/LConn2 -- RG4in/RConn2
  108-300 3/RConn3 -- 300/LConn3
  107 Y PQ/LConn1 -- 107/RConn1
  SSN group tag19/LConn1 -- 61/RConn3 -- SSN9/LConn3
  106 Y PQ/LConn1 -- 106/RConn1 -- 106-107 10/LConn1
  450/LConn3 -- 100-450 3/RConn3
  110-111 9/LConn1 -- 111/LConn1
  113-114 9/RConn1 -- 114/LConn1
  102/LConn1 -- 101-102 11/RConn1
  XF1/LConn1 -- 61-610/RConn1
  109/LConn1 -- 108-109 9/RConn1
  Regulator 4/LConn3 -- RG4in/RConn3
  105/RConn3 -- 105-108 3/LConn3
  61/LConn1 -- 60-61 5/RConn1
  610/LConn3 -- Three-Phase Transformer (Two Windings)/RConn3
  105/RConn1 -- 105-108 3/LConn1
  112 Y I/LConn1 -- 112/RConn1 -- 112-113 9/LConn1
  Ground74/LConn1 -- 109 Y PQ/RConn1
  98 Y PQ/LConn1 -- 98/RConn1 -- 98-99 3/LConn1
  Ground78/LConn1 -- 142 Y PQ/RConn1
  300/RConn1 -- Load Flow Bus44/LConn1
  66/LConn2 -- 65-66 12/RConn2
  61-610/RConn3 -- XF1/LConn3
  300/RConn2 -- Load Flow Bus44/LConn2
  610/RConn2 -- Load Flow Bus84/LConn2
  160/RConn2 -- 160 67 6/LConn2
  SSN6/RConn2 -- 300-1/LConn2
  66/LConn1 -- 65-66 12/RConn1
  160/RConn1 -- 160 67 6/LConn1
  SSN9/LConn1 -- 61/RConn1
  67-97 3/LConn1 -- RG4out/RConn1 -- RG4outa/RConn1
  98/LConn2 -- 97-98 3/RConn2
  450/RConn1 -- Load Flow Bus106/LConn1
  SSN7/LConn1 -- Load Flow Bus106/RConn1
  97-1/LConn1 -- SSN8/LConn1
  99/LConn1 -- 98-99 3/RConn1
  97-1/LConn3 -- SSN8/LConn3
  300-1/RConn1 -- Load Flow Bus45/LConn1
  65/RConn3 -- 65-66 12/LConn3
  SSN7/RConn1 -- 450-451/LConn1
  99/RConn3 -- 99-100 3/LConn3
  60-1/RConn2 -- SSN10/LConn2
  SSN6/RConn1 -- 300-1/LConn1
  XF1/RConn2 -- Three-Phase Transformer (Two Windings)/LConn2
  300-1/RConn3 -- Load Flow Bus45/LConn3
  66/RConn2 -- Load Flow Bus128/LConn2
  Regulator 4/LConn1 -- RG4in/RConn1
  450-451/RConn2 -- Load Flow Bus107/LConn2
  SSN9/LConn2 -- 61/RConn2
  160/LConn1 -- SSN10/RConn1
  98/LConn1 -- 97-98 3/RConn1
  450/RConn3 -- Load Flow Bus106/LConn3
  Ground72/LConn1 -- 106 Y PQ/RConn1
  64/LConn3 -- 63-64 12/RConn3
  63/LConn3 -- 62-63 12/RConn3
  66/RConn1 -- Load Flow Bus128/LConn1
  197/LConn2 -- 97-1/RConn2
  114/RConn1 -- 142 Y PQ/LConn1
  107/LConn1 -- 106-107 10/RConn1
  64/RConn1 -- 64-65 12/LConn1
  610/RConn1 -- Load Flow Bus84/LConn1
  610/LConn2 -- Three-Phase Transformer (Two Windings)/RConn2
  450/LConn1 -- 100-450 3/RConn1
  104/LConn1 -- 103-104 11/RConn1
  66/LConn3 -- 65-66 12/RConn3
  610/RConn3 -- Load Flow Bus84/LConn3
  RG4in/LConn3 -- 160 67 6/RConn3
  Ground68/LConn1 -- 100 Y Z/RConn1
  XF1/LConn2 -- 61-610/RConn2
  RG4in/LConn2 -- 160 67 6/RConn2
  197/RConn2 -- 197-101 3/LConn2
  Regulator 4/RConn2 -- RG4out/LConn2
  113 Y Z/LConn1 -- 113/RConn1 -- 113-114 9/LConn1
  Regulator 4/RConn3 -- RG4out/LConn3
  100/LConn2 -- 99-100 3/RConn2
  60/RConn1 -- 60a/RConn1
  60/RConn3 -- 60c/RConn1
